simulink model "rfxolg29"  (Simulink 4.00)
settings: Solver=ode4  StartTime=0.0  StopTime=16  FixedStep=.004  MaxStep=0.1  MinStep=0.005  RelTol=1e-3  AbsTol=1e-3
settings Model: LastModifiedBy=arthur  SaveTime=off  SaveOutput=off

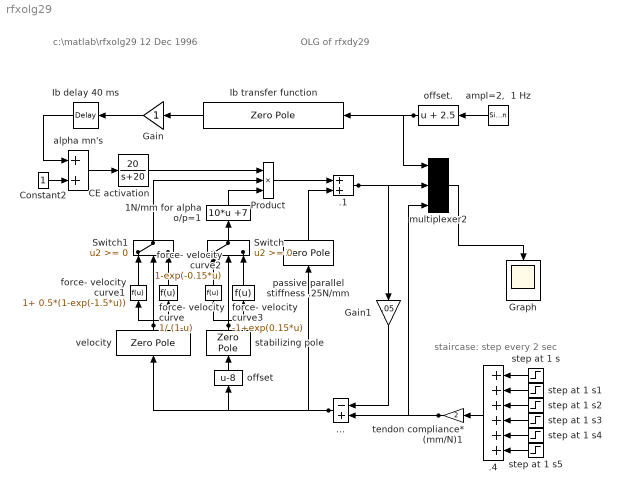
== system rfxolg29 ==
  note: OLG of rfxdy29
  note: c:\matlab\rfxolg29 12 Dec 1996
  note: staircase: step every 2 sec
  ... : Sum  Orientation=left  Inputs=-+  SaturateOnIntegerOverflow=on
  .1 : Sum  Inputs=++  SaturateOnIntegerOverflow=on
  .4 : Sum  Orientation=left  Inputs=++++++  SaturateOnIntegerOverflow=on
  1N/mm for alpha o/p=1 : Fcn  Orientation=up  Expr=10*u +7
  CE activation : TransferFcn  Numerator=[20]  Denominator=[1 20]  AbsoluteTolerance=auto  Realization=auto
  Constant2 : Constant  Value=1
  Gain : Gain  Orientation=left  Gain=1  Multiplication=Element-wise(K.*u)  SaturateOnIntegerOverflow=on
  Gain1 : Gain  Orientation=down  Gain=.05  Multiplication=Element-wise(K.*u)  SaturateOnIntegerOverflow=on
  Graph : Scope
      settings: Orientation=down  TimeRange=16  YMin=0  YMax=30  SaveToWorkspace=off  DataFormat=Array  LimitDataPoints=on  MaxDataPoints=5000
  Ib delay 40 ms : TransportDelay  Orientation=left  DelayTime=.04  InitialInput=0  BufferSize=1024  PadeOrder=0
  Ib transfer function : ZeroPole  Orientation=left  Zeros=[-.15; -1.5; -16]  Poles=[-.2; -2; -37]  Gain=[.28]  AbsoluteTolerance=auto
  Product : Product  Inputs=3  Multiplication=Element-wise(.*)  SaturateOnIntegerOverflow=on
  Switch : Switch  Orientation=up  Threshold=0
  Switch1 : Switch  Orientation=up  Threshold=0
  alpha mn's : Sum  Inputs=++  SaturateOnIntegerOverflow=on
  "ampl=2,  1 Hz " : SignalGenerator  Orientation=left  WaveForm=sine  Amplitude=2.500000  Frequency=6.280000  Units=rad/sec
  force- velocity curve : Fcn  Orientation=up  Expr=1/ (1-u)
  force- velocity curve1 : Fcn  Orientation=up  Expr=1+ 0.5*(1-exp(-1.5*u))
  force- velocity curve2 : Fcn  Orientation=up  Expr=1-exp(-0.15*u)
  force- velocity curve3 : Fcn  Orientation=up  Expr=-1+exp(0.15*u)
  multiplexer2 : Mux  Inputs=3
      settings: DisplayOption=none
  offset : Fcn  Orientation=up  Expr=u-8
  offset. : Fcn  Orientation=left  Expr=u + 2.5
  passive parallel stiffness .25N/mm : ZeroPole  Orientation=up  Zeros=[-25]  Poles=[-1000]  Gain=[10]  AbsoluteTolerance=auto
  stabilizing pole : ZeroPole  Orientation=up  Zeros=[ ]  Poles=[-100]  Gain=[100]  AbsoluteTolerance=auto
  step at 1 s : Step  Orientation=left  Time=2  Before=0  After=1  SampleTime=-1
  step at 1 s1 : Step  Orientation=left  Time=4  Before=0  After=1  SampleTime=-1
  step at 1 s2 : Step  Orientation=left  Time=6  Before=0  After=1  SampleTime=-1
  step at 1 s3 : Step  Orientation=left  Time=8  Before=0  After=1  SampleTime=-1
  step at 1 s4 : Step  Orientation=left  Time=10  Before=0  After=1  SampleTime=-1
  step at 1 s5 : Step  Orientation=left  Time=12  Before=0  After=1  SampleTime=-1
  tendon compliance* (mm/N)1 : Gain  Orientation=left  Gain=2  Multiplication=Element-wise(K.*u)  SaturateOnIntegerOverflow=on
      settings: OpenFcn=slideg(0,2,10,0)
      mask Display: disp('2')
  velocity : ZeroPole  Orientation=up  Zeros=[0]  Poles=[-100;-100]  Gain=[150]  AbsoluteTolerance=auto
  wires:
  Gain/1 -> Ib delay 40 ms/1
  alpha mn's/1 -> CE activation/1
  Ib delay 40 ms/1 -> alpha mn's/1
  Product/1 -> .1/1
  CE activation/1 -> Product/1
  Constant2/1 -> alpha mn's/2
  passive parallel stiffness .25N/mm/1 -> .1/2
  .../1 -> offset/1, passive parallel stiffness .25N/mm/1, velocity/1
  Gain1/1 -> .../1
  .1/1 -> multiplexer2/2, Gain1/1
  offset./1 -> multiplexer2/1, Ib transfer function/1
  "ampl=2,  1 Hz "/1 -> offset./1
  Ib transfer function/1 -> Gain/1
  step at 1 s/1 -> .4/1
  step at 1 s1/1 -> .4/2
  step at 1 s2/1 -> .4/3
  step at 1 s3/1 -> .4/4
  step at 1 s4/1 -> .4/5
  step at 1 s5/1 -> .4/6
  .4/1 -> tendon compliance* (mm/N)1/1
  tendon compliance* (mm/N)1/1 -> .../2, multiplexer2/3
  multiplexer2/1 -> Graph/1
  offset/1 -> stabilizing pole/1
  stabilizing pole/1 -> Switch/2, force- velocity curve3/1, force- velocity curve2/1
  force- velocity curve3/1 -> Switch/3
  force- velocity curve2/1 -> Switch/1
  Switch/1 -> 1N/mm for alpha o/p=1/1
  force- velocity curve/1 -> Switch1/3
  force- velocity curve1/1 -> Switch1/1
  velocity/1 -> Switch1/2, force- velocity curve/1, force- velocity curve1/1
  Switch1/1 -> Product/2
  1N/mm for alpha o/p=1/1 -> Product/3
